simulink model "Wo_bu_zhidao_Simulink_de_guanxi"  (R2015b)
settings: Solver=FixedStepDiscrete  StartTime=0.0  StopTime=inf  FixedStep=1  RelTol=1e-3
libraries: instrumentlib x1, simulink x1
settings Model: Creator=ykwo675  LastModifiedBy=ykwo675
settings SolverCC: AutoInsertRateTranBlk=on

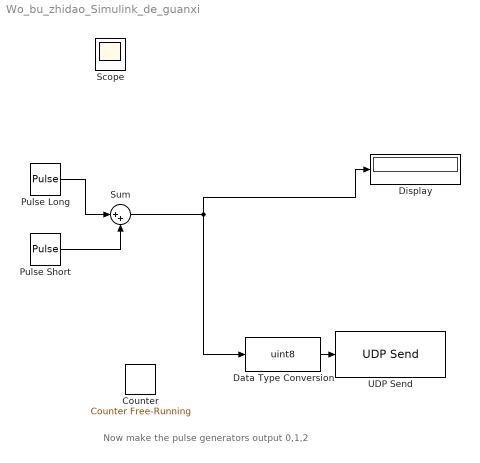
== system Wo_bu_zhidao_Simulink_de_guanxi ==
  note: Now make the pulse generators output 0,1,2
  Data Type Conversion : DataTypeConversion  OutDataTypeStr=uint8
  Display : Display
  Pulse Long : DiscretePulseGenerator  PulseType=Time based  Period=20000  PulseWidth=50
  Pulse Short : DiscretePulseGenerator  PulseType=Time based  Period=10000  PulseWidth=50
  Sum : Sum  Inputs=|++
  UDP Send : instrumentlib/UDP Send  Host=127.0.0.1  Port=1111  LocalPort=-1  EnableBlockingMode=on  ByteOrder=BigEndian
  "Counter " : simulink/Sources/Counter Free-Running  IOType=siggen  NumBits=16  tsamp=-1
  Scope : Scope
  wires:
  Sum/1 -> Display/1, Data Type Conversion/1
  Data Type Conversion/1 -> UDP Send/1
  Pulse Long/1 -> Sum/1
  Pulse Short/1 -> Sum/2
